simulink model "VV_Graph_all"  (R2018b)
settings: Solver=FixedStepAuto  StartTime=0.0  StopTime=10.0  FixedStep=0.001  RelTol=1e-3
settings Model: Creator=kekos  LastModifiedBy=kekos

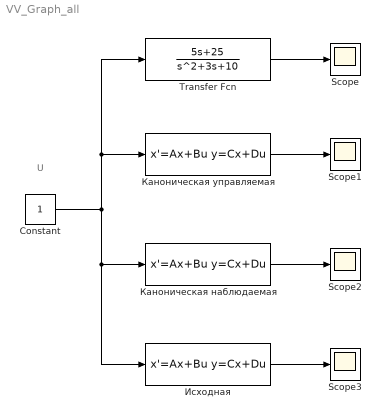
== system VV_Graph_all ==
  note: U
  Constant : Constant
  Scope{,1..3} (4 alike) : Scope
  Transfer Fcn : TransferFcn  Numerator=[5 25]  Denominator=[1 3 10]
  Исходная : StateSpace  A=[0 2; -5 -3]  B=[1; 1]  C=[5 0]  InitialCondition=0
  Каноническая наблюдаемая : StateSpace  A=[0 -10; 1 -3]  B=[25; 5]  C=[0 1]  InitialCondition=0
  Каноническая управляемая : StateSpace  A=[0 1; -10 -3]  B=[0; 1;]  C=[25 5]  InitialCondition=0
  wires:
  Каноническая наблюдаемая/1 -> Scope2/1
  Constant/1 -> Transfer Fcn/1, Каноническая управляемая/1, Исходная/1, Каноническая наблюдаемая/1
  Каноническая управляемая/1 -> Scope1/1
  Transfer Fcn/1 -> Scope/1
  Исходная/1 -> Scope3/1
